simulink model "wtgtest"  (R2021a)
settings: Solver=VariableStepAuto  StartTime=0.0  StopTime=10.0  RelTol=1e-3
undefined symbols (not defined in the file or in its folder): deg, rad, s
libraries: aerolibconvert2 x1
settings Model: Creator=Chitra Manis Raja  LastModifiedBy=Chitra Manis Raja

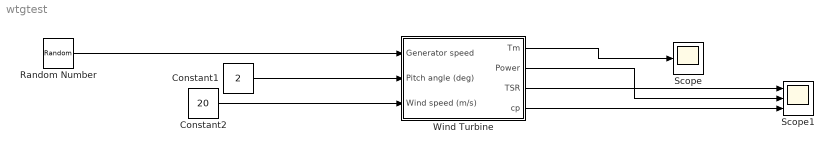
== system wtgtest ==
  Constant1 : Constant  Value=2
  Constant2 : Constant  Value=20
  Random Number : RandomNumber  Mean=12  SampleTime=0.1
  Scope : Scope
  Scope1 : Scope  NumInputPorts=3
  Wind Turbine : Subsystem  AncestorBlock=spsWindTurbineLib/Wind Turbine  DialogController=POWERSYS.PowerSysDialog  mask(Wind Turbine){Pnom=1.5e6, Pelec_base=1.5e6/0.9, wind_base=12, P_wind_base=0.73, speed_nom=1.2, pitch_angle=0, c1_c6=[0.51763          116          0.4            5           21     0.006795], cp_nom=0.48, lambda_nom=8.1}
      mask prompts: Pnom "Nominal mechanical output power (W):"; Pelec_base "Base power of the electrical generator (VA):"; wind_base "Base wind speed (m/s):"; P_wind_base "Maximum power at base wind speed (pu of nominal mechanical power):"; speed_nom "Base rotational speed (p.u. of base generator speed):"; pitch_angle "Pitch angle beta to display wind-turbine power characteristics (beta >=0)  (deg):"
      mask help:
      | This block implements a variable pitch wind turbine model. The performance coefficient Cp of the turbine is the mechanical output power of the turbine divided by wind power and a function of wind speed, rotational speed, and pitch angle (beta). Cp reaches its maximum value at zero beta. Select the wind-turbine power characteristics display to plot the turbine characteristics at the specified pitch angle.
      |
      | The first input is the generator speed in per unit of the generator base speed. For a synchronous or asynchronous generator, the base speed is the synchronous speed. For a permanent-magnet generator, the base speed is defined as the speed producing nominal voltage at  no load. The second input is the blade pitch angle (beta) in degrees. The third input is the wind speed in m/s.
      |
      | The output is the torque applied to the generator shaft in per unit of the generator ratings.
      |
      | The turbine inertia must be added to the generator inertia.
      mask init:
      | c1=c1_c6(1);c2=c1_c6(2);c3=c1_c6(3);c4=c1_c6(4);c5=c1_c6(5);c6=c1_c6(6);
      | 
      | if Pnom<=0
      |     error(message('physmod:powersys:common:GreaterThan',getfullname(gcbh),'Nominal mechanical output power',0));
      | end
      | if Pelec_base<=0
      |     error(message('physmod:powersys:common:GreaterThan',getfullname(gcbh),'Base power of the electrical generator',0));
      | end
      | if wind_base<=0
      |     error(message('physmod:powersys:common:GreaterThan',getfullname(gcbh),'Base wind speed (m/s)',0));
      | end
      | if P_wind_base<=0
      |     error(message('physmod:powersys:common:GreaterThan',getfullname(gcbh),'Maximum power at base wind speed',0));
      | end
      | power_initmask();
      settings: OpenFcn=sps_rtmsupport('OpenFcn',gcbh)
      mask Help: helpview(psbhelp);
      mask DialogControl DisplayTurbChar Prompt: Display wind turbine power characteristics
      mask DialogControl DisplayTurbChar Callback: WindTurbinePlot(gcb)
  wires:
  Random Number/1 -> Wind Turbine/1(Generator speed)
  Constant1/1 -> Wind Turbine/2(Pitch angle (deg))
  Constant2/1 -> Wind Turbine/3(Wind speed (m/s))
  Wind Turbine/1("Tm ") -> Scope/1
  Wind Turbine/2(Power) -> Scope1/2
  Wind Turbine/3(TSR) -> Scope1/1
  Wind Turbine/4(cp) -> Scope1/3

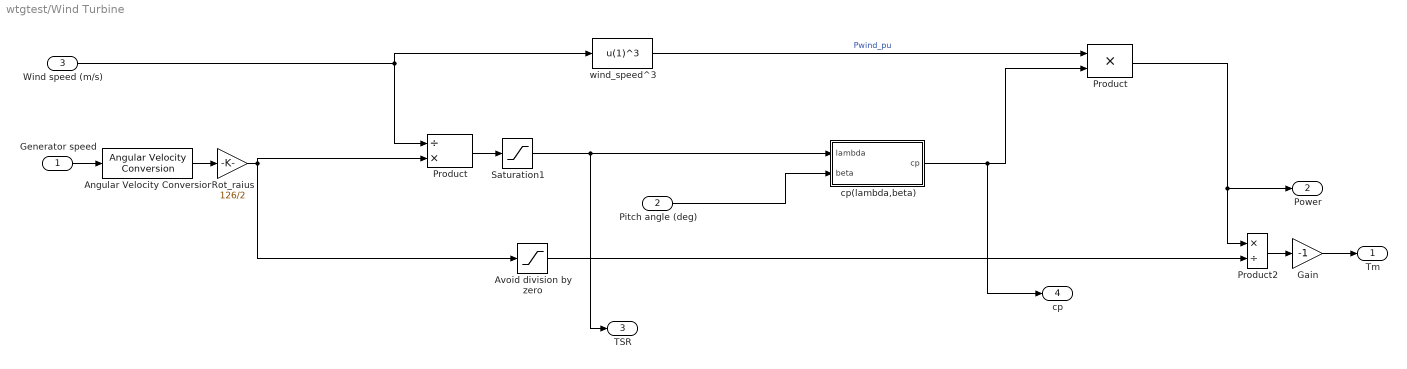
== system wtgtest/Wind Turbine ==
  Generator speed : Inport
  Pitch angle (deg) : Inport  Port=2
  Wind speed (m/s) : Inport  Port=3
  Angular Velocity Conversion : aerolibconvert2/Angular Velocity Conversion  IU=deg/s  OU=rad/s
  Avoid division by zero : Saturate  UpperLimit=1e6  LowerLimit=1e-6
  Gain : Gain  Gain=-1  SaturateOnIntegerOverflow=on  OutDataTypeStr=Inherit: Same as input  ParamDataTypeStr=Inherit: Same as input
  Product : Product  Inputs=/*  SaturateOnIntegerOverflow=on  OutDataTypeStr=Inherit: Same as first input
  "Product " : Product  SaturateOnIntegerOverflow=on  OutDataTypeStr=Inherit: Same as first input
  Product2 : Product  Inputs=*/  InputSameDT=on  SaturateOnIntegerOverflow=on  OutDataTypeStr=Inherit: Same as first input
  Rot_raius : Gain  Gain=126/2
  Saturation1 : Saturate  UpperLimit=inf  LowerLimit=1e-6
  cp(lambda,beta) : Subsystem
  wind_speed^3 : Fcn  Expr=u(1)^3
  "Tm " : Outport  VectorParamsAs1DForOutWhenUnconnected=off
  Power : Outport  Port=2
  TSR : Outport  Port=3
  cp : Outport  Port=4
  wires:
  Pitch angle (deg)/1 -> cp(lambda,beta)/2(beta)
  wind_speed^3/1 -> "Product "/1  "Pwind_pu"
  Product2/1 -> Gain/1
  Avoid division by zero/1 -> Product2/2
  Gain/1 -> "Tm "/1
  Saturation1/1 -> TSR/1, cp(lambda,beta)/1(lambda)
  Wind speed (m/s)/1 -> Product/1, wind_speed^3/1
  Product/1 -> Saturation1/1
  cp(lambda,beta)/1(cp) -> cp/1, "Product "/2
  "Product "/1 -> Power/1, Product2/1
  Generator speed/1 -> Angular Velocity Conversion/1
  Angular Velocity Conversion/1 -> Rot_raius/1
  Rot_raius/1 -> Avoid division by zero/1, Product/2

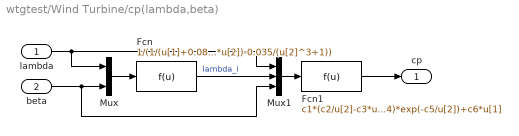
== system wtgtest/Wind Turbine/cp(lambda,beta) ==
  lambda : Inport
  beta : Inport  Port=2
  Fcn : Fcn  Expr=1/(1/(u[1]+0.08*u[2])-0.035/(u[2]^3+1))
  Fcn1 : Fcn  Expr=c1*(c2/u[2]-c3*u[3]-c4)*exp(-c5/u[2])+c6*u[1]
  Mux : Mux  Inputs=2
  Mux1 : Mux  Inputs=3
  cp : Outport  VectorParamsAs1DForOutWhenUnconnected=off
  wires:
  Fcn/1 -> Mux1/2  "lambda_i"
  Fcn1/1 -> cp/1
  lambda/1 -> Mux1/1, Mux/1
  Mux1/1 -> Fcn1/1
  beta/1 -> Mux1/3, Mux/2
  Mux/1 -> Fcn/1
